simulink model "npc_controller"  (R2022a)
settings: Solver=FixedStepDiscrete  StartTime=0.0  StopTime=20  RelTol=1e-3  EnableMultiTasking=on
undefined symbols (not defined in the file): CAN_O_INT, CANA_BASE, Down, GPTRIP1SEL, GPTRIP2SEL, GPTRIP3SEL, Tsw, TZ1, TZ2, TZ3, Up, V2G_en
libraries: simulink x171, hdlsllib x90, c2802xlib x46, c2837xDlib x19, c280xlib x12, canmsglib x9, c2838xlib x8, idelinklib_common x5, c2806xlib x2, slpidlib x2, c28004xlib x2, c281xlib x2
(part 50 of 55)

== system npc_controller/IDLE_AND_TIMER/codegen/CAN_Task/Tx_Handler/Run Tx Routine/TxStatusData/Tx Pri2 ID131 ==
  Action Port : ActionPort  ActionPortLabel=case [ 2 ]:
  CAN Pack1 : canmsglib/CAN Pack  MsgList=(none)  MsgName=CAN Msg  MsgIDType=Standard (11-bit identifier)  MsgIdentifier=0x131  MsgLength=8  Remote=off  ApplyMinMax=off  BusOutput=off  SignalInfo={}
      settings: SourceProductBaseCode=XP,ME,VN  DataFormat=raw data
  Constant1 : Constant  Value=3  OutDataTypeStr=uint8
  Constant2 : Constant  Value=0.1  OutDataTypeStr=single
  Constant3 : Constant  Value=0.01  OutDataTypeStr=single
  Constant4 : Constant  Value=0.01  OutDataTypeStr=single
  Constant5 : Constant  Value=0.1  OutDataTypeStr=single
  Data Store Read1 : DataStoreRead  DataStoreName=f32VinB  IndexOptions=Index vector (dialog)  Indices=1  OutputSizes=1
  Data Store Read2 : DataStoreRead  DataStoreName=f32VinC  IndexOptions=Index vector (dialog)  Indices=1  OutputSizes=1
  Data Store Read4 : DataStoreRead  DataStoreName=f32IinB  IndexOptions=Index vector (dialog)  Indices=1  OutputSizes=1
  Data Store Read5 : DataStoreRead  DataStoreName=f32IinC  IndexOptions=Index vector (dialog)  Indices=1  OutputSizes=1
  Data Store Write1 : DataStoreWrite  DataStoreName=u8CanTxIndex  IndexOptions=Index vector (dialog)  Indices=1  OutputSizes=1
  Float Data to Bytes : Subsystem
  Float Data to Bytes1 : Subsystem
  Float Data to Bytes2 : Subsystem
  Float Data to Bytes3 : Subsystem
  Vector Concatenate : Concatenate  NumInputs=8
  eCAN Transmit : c280xlib/eCAN Transmit  chipFamily=C280x  useModule=eCAN_A  mailboxNo=2  messageID=hex2dec('0131')  messageType=Standard (11-bit identifier)  enableBlockingMode=off  postInterrupt=off  interruptLine=0
      settings: SourceProductBaseCode=TIC2000
  wires:
  Constant1/1 -> Data Store Write1/1
  Data Store Read4/1 -> Float Data to Bytes1/1(Float Data)
  Data Store Read2/1 -> Float Data to Bytes/1(Float Data)
  Constant2/1 -> Float Data to Bytes/2(Resol.)
  CAN Pack1/1 -> eCAN Transmit/1
  Float Data to Bytes/1(u8Lsb) -> Vector Concatenate/3
  Float Data to Bytes3/1(u8Lsb) -> Vector Concatenate/1
  Float Data to Bytes3/2(u8Msb) -> Vector Concatenate/2
  Float Data to Bytes2/2(u8Msb) -> Vector Concatenate/8
  Constant4/1 -> Float Data to Bytes2/2(Resol.)
  Float Data to Bytes2/1(u8Lsb) -> Vector Concatenate/7
  Data Store Read5/1 -> Float Data to Bytes2/1(Float Data)
  Float Data to Bytes/2(u8Msb) -> Vector Concatenate/4
  Data Store Read1/1 -> Float Data to Bytes3/1(Float Data)
  Float Data to Bytes1/1(u8Lsb) -> Vector Concatenate/5
  Vector Concatenate/1 -> CAN Pack1/1
  Constant3/1 -> Float Data to Bytes1/2(Resol.)
  Float Data to Bytes1/2(u8Msb) -> Vector Concatenate/6
  Constant5/1 -> Float Data to Bytes3/2(Resol.)

== system npc_controller/IDLE_AND_TIMER/codegen/CAN_Task/Tx_Handler/Run Tx Routine/TxStatusData/Tx Pri3 ID132 ==
  Action Port : ActionPort  ActionPortLabel=case [ 3 ]:
  CAN Pack1 : canmsglib/CAN Pack  MsgList=(none)  MsgName=CAN Msg  MsgIDType=Standard (11-bit identifier)  MsgIdentifier=0x132  MsgLength=8  Remote=off  ApplyMinMax=off  BusOutput=off  SignalInfo={}
      settings: SourceProductBaseCode=XP,ME,VN  DataFormat=raw data
  Constant1 : Constant  Value=4  OutDataTypeStr=uint8
  Constant2 : Constant  Value=0.01  OutDataTypeStr=single
  Constant3 : Constant  Value=0.01  OutDataTypeStr=single
  Constant4 : Constant  Value=0.1  OutDataTypeStr=single
  Constant5 : Constant  Value=0.01  OutDataTypeStr=single
  Data Store Read1 : DataStoreRead  DataStoreName=f32IphaseA  IndexOptions=Index vector (dialog)  Indices=1  OutputSizes=1
  Data Store Read2 : DataStoreRead  DataStoreName=f32IphaseB  IndexOptions=Index vector (dialog)  Indices=1  OutputSizes=1
  Data Store Read4 : DataStoreRead  DataStoreName=f32IphaseC  IndexOptions=Index vector (dialog)  Indices=1  OutputSizes=1
  Data Store Read5 : DataStoreRead  DataStoreName=f32Vpfc  IndexOptions=Index vector (dialog)  Indices=1  OutputSizes=1
  Data Store Write1 : DataStoreWrite  DataStoreName=u8CanTxIndex  IndexOptions=Index vector (dialog)  Indices=1  OutputSizes=1
  Float Data to Bytes : Subsystem
  Float Data to Bytes1 : Subsystem
  Float Data to Bytes2 : Subsystem
  Float Data to Bytes3 : Subsystem
  Vector Concatenate : Concatenate  NumInputs=8
  eCAN Transmit : c280xlib/eCAN Transmit  chipFamily=C280x  useModule=eCAN_A  mailboxNo=2  messageID=hex2dec('0132')  messageType=Standard (11-bit identifier)  enableBlockingMode=off  postInterrupt=off  interruptLine=0
      settings: SourceProductBaseCode=TIC2000
  wires:
  Constant5/1 -> Float Data to Bytes3/2(Resol.)
  Float Data to Bytes1/2(u8Msb) -> Vector Concatenate/6
  Constant3/1 -> Float Data to Bytes1/2(Resol.)
  Vector Concatenate/1 -> CAN Pack1/1
  Float Data to Bytes1/1(u8Lsb) -> Vector Concatenate/5
  Data Store Read1/1 -> Float Data to Bytes3/1(Float Data)
  Float Data to Bytes/2(u8Msb) -> Vector Concatenate/4
  Data Store Read5/1 -> Float Data to Bytes2/1(Float Data)
  Float Data to Bytes2/1(u8Lsb) -> Vector Concatenate/7
  Constant4/1 -> Float Data to Bytes2/2(Resol.)
  Float Data to Bytes2/2(u8Msb) -> Vector Concatenate/8
  Float Data to Bytes3/2(u8Msb) -> Vector Concatenate/2
  Float Data to Bytes3/1(u8Lsb) -> Vector Concatenate/1
  Float Data to Bytes/1(u8Lsb) -> Vector Concatenate/3
  CAN Pack1/1 -> eCAN Transmit/1
  Constant2/1 -> Float Data to Bytes/2(Resol.)
  Data Store Read2/1 -> Float Data to Bytes/1(Float Data)
  Data Store Read4/1 -> Float Data to Bytes1/1(Float Data)
  Constant1/1 -> Data Store Write1/1

== system npc_controller/IDLE_AND_TIMER/codegen/CAN_Task/Tx_Handler/Run Tx Routine/TxStatusData/Tx Pri4 ID133 ==
  Action Port : ActionPort  ActionPortLabel=case [ 4 ]:
  CAN Pack1 : canmsglib/CAN Pack  MsgList=(none)  MsgName=CAN Msg  MsgIDType=Standard (11-bit identifier)  MsgIdentifier=0x133  MsgLength=8  Remote=off  ApplyMinMax=off  BusOutput=off  SignalInfo={}
      settings: SourceProductBaseCode=XP,ME,VN  DataFormat=raw data
  Constant1 : Constant  Value=0  OutDataTypeStr=uint8
  Constant2 : Constant  Value=0  OutDataTypeStr=uint8
  Data Store Read1 : DataStoreRead  DataStoreName=u8TnpcA  IndexOptions=Index vector (dialog)  Indices=1  OutputSizes=1
  Data Store Read2 : DataStoreRead  DataStoreName=u8TnpcC  IndexOptions=Index vector (dialog)  Indices=1  OutputSizes=1
  Data Store Read3 : DataStoreRead  DataStoreName=u8TnpcB  IndexOptions=Index vector (dialog)  Indices=1  OutputSizes=1
  Data Store Read4 : DataStoreRead  DataStoreName=u8TclllcP2  IndexOptions=Index vector (dialog)  Indices=1  OutputSizes=1
  Data Store Read6 : DataStoreRead  DataStoreName=u8TclllcP1  IndexOptions=Index vector (dialog)  Indices=1  OutputSizes=1
  Data Store Write1 : DataStoreWrite  DataStoreName=u8CanTxIndex  IndexOptions=Index vector (dialog)  Indices=1  OutputSizes=1
  Vector Concatenate : Concatenate  NumInputs=8
  eCAN Transmit : c280xlib/eCAN Transmit  chipFamily=C280x  useModule=eCAN_A  mailboxNo=3  messageID=hex2dec('0133')  messageType=Standard (11-bit identifier)  enableBlockingMode=off  postInterrupt=off  interruptLine=0
      settings: SourceProductBaseCode=TIC2000
  wires:
  Constant1/1 -> Data Store Write1/1
  CAN Pack1/1 -> eCAN Transmit/1
  Data Store Read1/1 -> Vector Concatenate/1
  Data Store Read3/1 -> Vector Concatenate/2
  Vector Concatenate/1 -> CAN Pack1/1
  Data Store Read6/1 -> Vector Concatenate/4
  Data Store Read2/1 -> Vector Concatenate/3
  Data Store Read4/1 -> Vector Concatenate/5
  Constant2/1 -> Vector Concatenate/6, Vector Concatenate/7, Vector Concatenate/8

== system npc_controller/IDLE_AND_TIMER/codegen/IDLE/idle_task/hkeep/tfv/hkeep1/HKEEP.tfvIphaseA ==
  input : Inport  OutDataTypeStr=uint16  PortDimensions=1
  assert_lim : Inport  Port=2  OutDataTypeStr=uint16  PortDimensions=1
  assert_vld : Inport  Port=3  OutDataTypeStr=uint16  PortDimensions=1
  deassert_lim : Inport  Port=4  OutDataTypeStr=uint16  PortDimensions=1
  deassert_vld : Inport  Port=5  OutDataTypeStr=uint16  PortDimensions=1
  f : TriggerPort  TriggerType=function-call  VariantControl=(inherit)
      settings: CopyFcn=Stateflow.SLINSF.SimulinkMan.removeBlockPreDeleteFcn  PreDeleteFcn=Stateflow.SLINSF.SimulinkMan.unsafePredeleteFcn
  Data Store Read : DataStoreRead  DataStoreName=cnt_1ms  IndexOptions=Index vector (dialog)  Indices=1  OutputSizes=1
  Data Type Conversion : DataTypeConversion  OutDataTypeStr=boolean  SaturateOnIntegerOverflow=off  RndMeth=Floor
  MATLAB System : MATLABSystem  System=tfv_latch  SimulateUsing=Code generation
      mask Type: tfv_latch
      mask Display:
      | disp('tfv_latch');
      | port_label('input',1,'input');
      | port_label('input',2,'assert_lim');
      | port_label('input',3,'assert_vld');
      | port_label('input',4,'deassert_lim');
      | port_label('input',5,'deassert_vld');
      | port_label('input',6,'tmr');
      | port_label('output',1,'status');
  tfv_iphasaea : Outport  OutDataTypeStr=boolean
  wires:
  Data Type Conversion/1 -> tfv_iphasaea/1
  Data Store Read/1 -> MATLAB System/6
  deassert_vld/1 -> MATLAB System/5
  deassert_lim/1 -> MATLAB System/4
  assert_vld/1 -> MATLAB System/3
  assert_lim/1 -> MATLAB System/2
  input/1 -> MATLAB System/1
  MATLAB System/1 -> Data Type Conversion/1

== system npc_controller/IDLE_AND_TIMER/codegen/IDLE/idle_task/hkeep/tfv/hkeep1/HKEEP.tfvIphaseB ==
  input : Inport  OutDataTypeStr=uint16  PortDimensions=1
  assert_lim : Inport  Port=2  OutDataTypeStr=uint16  PortDimensions=1
  assert_vld : Inport  Port=3  OutDataTypeStr=uint16  PortDimensions=1
  deassert_lim : Inport  Port=4  OutDataTypeStr=uint16  PortDimensions=1
  deassert_vld : Inport  Port=5  OutDataTypeStr=uint16  PortDimensions=1
  f : TriggerPort  TriggerType=function-call  VariantControl=(inherit)
      settings: CopyFcn=Stateflow.SLINSF.SimulinkMan.removeBlockPreDeleteFcn  PreDeleteFcn=Stateflow.SLINSF.SimulinkMan.unsafePredeleteFcn
  Data Store Read : DataStoreRead  DataStoreName=cnt_1ms  IndexOptions=Index vector (dialog)  Indices=1  OutputSizes=1
  Data Type Conversion : DataTypeConversion  OutDataTypeStr=boolean  SaturateOnIntegerOverflow=off  RndMeth=Floor
  MATLAB System : MATLABSystem  System=tfv_latch  SimulateUsing=Code generation
      mask Type: tfv_latch
      mask Display:
      | disp('tfv_latch');
      | port_label('input',1,'input');
      | port_label('input',2,'assert_lim');
      | port_label('input',3,'assert_vld');
      | port_label('input',4,'deassert_lim');
      | port_label('input',5,'deassert_vld');
      | port_label('input',6,'tmr');
      | port_label('output',1,'status');
  tfv_iphaseb : Outport  OutDataTypeStr=boolean
  wires:
  Data Type Conversion/1 -> tfv_iphaseb/1
  Data Store Read/1 -> MATLAB System/6
  deassert_vld/1 -> MATLAB System/5
  deassert_lim/1 -> MATLAB System/4
  assert_vld/1 -> MATLAB System/3
  assert_lim/1 -> MATLAB System/2
  input/1 -> MATLAB System/1
  MATLAB System/1 -> Data Type Conversion/1

== system npc_controller/IDLE_AND_TIMER/codegen/IDLE/idle_task/hkeep/tfv/hkeep1/HKEEP.tfvIphaseC ==
  input : Inport  OutDataTypeStr=uint16  PortDimensions=1
  assert_lim : Inport  Port=2  OutDataTypeStr=uint16  PortDimensions=1
  assert_vld : Inport  Port=3  OutDataTypeStr=uint16  PortDimensions=1
  deassert_lim : Inport  Port=4  OutDataTypeStr=uint16  PortDimensions=1
  deassert_vld : Inport  Port=5  OutDataTypeStr=uint16  PortDimensions=1
  f : TriggerPort  TriggerType=function-call  VariantControl=(inherit)
      settings: CopyFcn=Stateflow.SLINSF.SimulinkMan.removeBlockPreDeleteFcn  PreDeleteFcn=Stateflow.SLINSF.SimulinkMan.unsafePredeleteFcn
  Data Store Read : DataStoreRead  DataStoreName=cnt_1ms  IndexOptions=Index vector (dialog)  Indices=1  OutputSizes=1
  Data Type Conversion : DataTypeConversion  OutDataTypeStr=boolean  SaturateOnIntegerOverflow=off  RndMeth=Floor
  MATLAB System : MATLABSystem  System=tfv_latch  SimulateUsing=Code generation
      mask Type: tfv_latch
      mask Display:
      | disp('tfv_latch');
      | port_label('input',1,'input');
      | port_label('input',2,'assert_lim');
      | port_label('input',3,'assert_vld');
      | port_label('input',4,'deassert_lim');
      | port_label('input',5,'deassert_vld');
      | port_label('input',6,'tmr');
      | port_label('output',1,'status');
  tfv_iphasec : Outport  OutDataTypeStr=boolean
  wires:
  Data Type Conversion/1 -> tfv_iphasec/1
  Data Store Read/1 -> MATLAB System/6
  deassert_vld/1 -> MATLAB System/5
  deassert_lim/1 -> MATLAB System/4
  assert_vld/1 -> MATLAB System/3
  assert_lim/1 -> MATLAB System/2
  input/1 -> MATLAB System/1
  MATLAB System/1 -> Data Type Conversion/1

== system npc_controller/IDLE_AND_TIMER/codegen/IDLE/idle_task/hkeep/tfv/hkeep1/HKEEP.tfvVa ==
  input : Inport  OutDataTypeStr=uint16  PortDimensions=1
  assert_lim : Inport  Port=2  OutDataTypeStr=uint16  PortDimensions=1
  assert_vld : Inport  Port=3  OutDataTypeStr=uint16  PortDimensions=1
  deassert_lim : Inport  Port=4  OutDataTypeStr=uint16  PortDimensions=1
  deassert_vld : Inport  Port=5  OutDataTypeStr=uint16  PortDimensions=1
  f : TriggerPort  TriggerType=function-call  VariantControl=(inherit)
      settings: CopyFcn=Stateflow.SLINSF.SimulinkMan.removeBlockPreDeleteFcn  PreDeleteFcn=Stateflow.SLINSF.SimulinkMan.unsafePredeleteFcn
  Data Store Read : DataStoreRead  DataStoreName=cnt_1ms  IndexOptions=Index vector (dialog)  Indices=1  OutputSizes=1
  Data Type Conversion : DataTypeConversion  OutDataTypeStr=boolean  SaturateOnIntegerOverflow=off  RndMeth=Floor
  MATLAB System : MATLABSystem  System=tfv_latch  SimulateUsing=Code generation
      mask Type: tfv_latch
      mask Display:
      | disp('tfv_latch');
      | port_label('input',1,'input');
      | port_label('input',2,'assert_lim');
      | port_label('input',3,'assert_vld');
      | port_label('input',4,'deassert_lim');
      | port_label('input',5,'deassert_vld');
      | port_label('input',6,'tmr');
      | port_label('output',1,'status');
  tfv_va : Outport  OutDataTypeStr=boolean
  wires:
  Data Type Conversion/1 -> tfv_va/1
  Data Store Read/1 -> MATLAB System/6
  deassert_vld/1 -> MATLAB System/5
  deassert_lim/1 -> MATLAB System/4
  assert_vld/1 -> MATLAB System/3
  assert_lim/1 -> MATLAB System/2
  input/1 -> MATLAB System/1
  MATLAB System/1 -> Data Type Conversion/1

== system npc_controller/IDLE_AND_TIMER/codegen/IDLE/idle_task/hkeep/tfv/hkeep1/HKEEP.tfvVaux ==
  input : Inport  OutDataTypeStr=uint16  PortDimensions=1
  assert_lim : Inport  Port=2  OutDataTypeStr=uint16  PortDimensions=1
  assert_vld : Inport  Port=3  OutDataTypeStr=uint16  PortDimensions=1
  deassert_lim : Inport  Port=4  OutDataTypeStr=uint16  PortDimensions=1
  deassert_vld : Inport  Port=5  OutDataTypeStr=uint16  PortDimensions=1
  f : TriggerPort  TriggerType=function-call  VariantControl=(inherit)
      settings: CopyFcn=Stateflow.SLINSF.SimulinkMan.removeBlockPreDeleteFcn  PreDeleteFcn=Stateflow.SLINSF.SimulinkMan.unsafePredeleteFcn
  Data Store Read : DataStoreRead  DataStoreName=cnt_1ms  IndexOptions=Index vector (dialog)  Indices=1  OutputSizes=1
  Data Type Conversion : DataTypeConversion  OutDataTypeStr=boolean  SaturateOnIntegerOverflow=off  RndMeth=Floor
  MATLAB System : MATLABSystem  System=tfv_latch  SimulateUsing=Code generation
      mask Type: tfv_latch
      mask Display:
      | disp('tfv_latch');
      | port_label('input',1,'input');
      | port_label('input',2,'assert_lim');
      | port_label('input',3,'assert_vld');
      | port_label('input',4,'deassert_lim');
      | port_label('input',5,'deassert_vld');
      | port_label('input',6,'tmr');
      | port_label('output',1,'status');
  Rate Transition2 : RateTransition  Commented=on
  tfv_vaux : Outport  OutDataTypeStr=boolean
  wires:
  Data Type Conversion/1 -> tfv_vaux/1
  deassert_vld/1 -> MATLAB System/5
  deassert_lim/1 -> MATLAB System/4
  assert_vld/1 -> MATLAB System/3
  assert_lim/1 -> MATLAB System/2
  input/1 -> MATLAB System/1
  MATLAB System/1 -> Data Type Conversion/1
  Data Store Read/1 -> MATLAB System/6

== system npc_controller/IDLE_AND_TIMER/codegen/IDLE/idle_task/hkeep/tfv/hkeep1/HKEEP.tfvVb ==
  input : Inport  OutDataTypeStr=uint16  PortDimensions=1
  assert_lim : Inport  Port=2  OutDataTypeStr=uint16  PortDimensions=1
  assert_vld : Inport  Port=3  OutDataTypeStr=uint16  PortDimensions=1
  deassert_lim : Inport  Port=4  OutDataTypeStr=uint16  PortDimensions=1
  deassert_vld : Inport  Port=5  OutDataTypeStr=uint16  PortDimensions=1
  f : TriggerPort  TriggerType=function-call  VariantControl=(inherit)
      settings: CopyFcn=Stateflow.SLINSF.SimulinkMan.removeBlockPreDeleteFcn  PreDeleteFcn=Stateflow.SLINSF.SimulinkMan.unsafePredeleteFcn
  Data Store Read : DataStoreRead  DataStoreName=cnt_1ms  IndexOptions=Index vector (dialog)  Indices=1  OutputSizes=1
  Data Type Conversion : DataTypeConversion  OutDataTypeStr=boolean  SaturateOnIntegerOverflow=off  RndMeth=Floor
  MATLAB System : MATLABSystem  System=tfv_latch  SimulateUsing=Code generation
      mask Type: tfv_latch
      mask Display:
      | disp('tfv_latch');
      | port_label('input',1,'input');
      | port_label('input',2,'assert_lim');
      | port_label('input',3,'assert_vld');
      | port_label('input',4,'deassert_lim');
      | port_label('input',5,'deassert_vld');
      | port_label('input',6,'tmr');
      | port_label('output',1,'status');
  tfv_vb : Outport  OutDataTypeStr=boolean
  wires:
  Data Type Conversion/1 -> tfv_vb/1
  Data Store Read/1 -> MATLAB System/6
  deassert_vld/1 -> MATLAB System/5
  deassert_lim/1 -> MATLAB System/4
  assert_vld/1 -> MATLAB System/3
  assert_lim/1 -> MATLAB System/2
  input/1 -> MATLAB System/1
  MATLAB System/1 -> Data Type Conversion/1

== system npc_controller/IDLE_AND_TIMER/codegen/IDLE/idle_task/hkeep/tfv/hkeep1/HKEEP.tfvVbulk ==
  input : Inport  OutDataTypeStr=uint16  PortDimensions=1
  assert_lim : Inport  Port=2  OutDataTypeStr=uint16  PortDimensions=1
  assert_vld : Inport  Port=3  OutDataTypeStr=uint16  PortDimensions=1
  deassert_lim : Inport  Port=4  OutDataTypeStr=uint16  PortDimensions=1
  deassert_vld : Inport  Port=5  OutDataTypeStr=uint16  PortDimensions=1
  f : TriggerPort  TriggerType=function-call  VariantControl=(inherit)
      settings: CopyFcn=Stateflow.SLINSF.SimulinkMan.removeBlockPreDeleteFcn  PreDeleteFcn=Stateflow.SLINSF.SimulinkMan.unsafePredeleteFcn
  Data Store Read : DataStoreRead  DataStoreName=cnt_1ms  IndexOptions=Index vector (dialog)  Indices=1  OutputSizes=1
  Data Type Conversion : DataTypeConversion  OutDataTypeStr=boolean  SaturateOnIntegerOverflow=off  RndMeth=Floor
  MATLAB System : MATLABSystem  System=tfv_latch  SimulateUsing=Code generation
      mask Type: tfv_latch
      mask Display:
      | disp('tfv_latch');
      | port_label('input',1,'input');
      | port_label('input',2,'assert_lim');
      | port_label('input',3,'assert_vld');
      | port_label('input',4,'deassert_lim');
      | port_label('input',5,'deassert_vld');
      | port_label('input',6,'tmr');
      | port_label('output',1,'status');
  tfv_vbulk : Outport  OutDataTypeStr=boolean
  wires:
  Data Type Conversion/1 -> tfv_vbulk/1
  Data Store Read/1 -> MATLAB System/6
  deassert_vld/1 -> MATLAB System/5
  deassert_lim/1 -> MATLAB System/4
  assert_vld/1 -> MATLAB System/3
  assert_lim/1 -> MATLAB System/2
  input/1 -> MATLAB System/1
  MATLAB System/1 -> Data Type Conversion/1

== system npc_controller/IDLE_AND_TIMER/codegen/IDLE/idle_task/hkeep/tfv/hkeep1/HKEEP.tfvVc ==
  input : Inport  OutDataTypeStr=uint16  PortDimensions=1
  assert_lim : Inport  Port=2  OutDataTypeStr=uint16  PortDimensions=1
  assert_vld : Inport  Port=3  OutDataTypeStr=uint16  PortDimensions=1
  deassert_lim : Inport  Port=4  OutDataTypeStr=uint16  PortDimensions=1
  deassert_vld : Inport  Port=5  OutDataTypeStr=uint16  PortDimensions=1
  f : TriggerPort  TriggerType=function-call  VariantControl=(inherit)
      settings: CopyFcn=Stateflow.SLINSF.SimulinkMan.removeBlockPreDeleteFcn  PreDeleteFcn=Stateflow.SLINSF.SimulinkMan.unsafePredeleteFcn
  Data Store Read : DataStoreRead  DataStoreName=cnt_1ms  IndexOptions=Index vector (dialog)  Indices=1  OutputSizes=1
  Data Type Conversion : DataTypeConversion  OutDataTypeStr=boolean  SaturateOnIntegerOverflow=off  RndMeth=Floor
  MATLAB System : MATLABSystem  System=tfv_latch  SimulateUsing=Code generation
      mask Type: tfv_latch
      mask Display:
      | disp('tfv_latch');
      | port_label('input',1,'input');
      | port_label('input',2,'assert_lim');
      | port_label('input',3,'assert_vld');
      | port_label('input',4,'deassert_lim');
      | port_label('input',5,'deassert_vld');
      | port_label('input',6,'tmr');
      | port_label('output',1,'status');
  tfv_vc : Outport  OutDataTypeStr=boolean
  wires:
  Data Type Conversion/1 -> tfv_vc/1
  Data Store Read/1 -> MATLAB System/6
  deassert_vld/1 -> MATLAB System/5
  deassert_lim/1 -> MATLAB System/4
  assert_vld/1 -> MATLAB System/3
  assert_lim/1 -> MATLAB System/2
  input/1 -> MATLAB System/1
  MATLAB System/1 -> Data Type Conversion/1

== system npc_controller/IDLE_AND_TIMER/codegen/IDLE/idle_task/hkeep/tfv/hkeep1/HKEEP.tfvVmid ==
  input : Inport  OutDataTypeStr=uint16  PortDimensions=1
  assert_lim : Inport  Port=2  OutDataTypeStr=uint16  PortDimensions=1
  assert_vld : Inport  Port=3  OutDataTypeStr=uint16  PortDimensions=1
  deassert_lim : Inport  Port=4  OutDataTypeStr=uint16  PortDimensions=1
  deassert_vld : Inport  Port=5  OutDataTypeStr=uint16  PortDimensions=1
  f : TriggerPort  TriggerType=function-call  VariantControl=(inherit)
      settings: CopyFcn=Stateflow.SLINSF.SimulinkMan.removeBlockPreDeleteFcn  PreDeleteFcn=Stateflow.SLINSF.SimulinkMan.unsafePredeleteFcn
  Data Store Read : DataStoreRead  DataStoreName=cnt_1ms  IndexOptions=Index vector (dialog)  Indices=1  OutputSizes=1
  Data Type Conversion : DataTypeConversion  OutDataTypeStr=boolean  SaturateOnIntegerOverflow=off  RndMeth=Floor
  MATLAB System : MATLABSystem  System=tfv_latch  SimulateUsing=Code generation
      mask Type: tfv_latch
      mask Display:
      | disp('tfv_latch');
      | port_label('input',1,'input');
      | port_label('input',2,'assert_lim');
      | port_label('input',3,'assert_vld');
      | port_label('input',4,'deassert_lim');
      | port_label('input',5,'deassert_vld');
      | port_label('input',6,'tmr');
      | port_label('output',1,'status');
  Rate Transition2 : RateTransition  Commented=on
  tfv_vmid : Outport  OutDataTypeStr=boolean
  wires:
  Data Type Conversion/1 -> tfv_vmid/1
  deassert_vld/1 -> MATLAB System/5
  deassert_lim/1 -> MATLAB System/4
  assert_vld/1 -> MATLAB System/3
  assert_lim/1 -> MATLAB System/2
  input/1 -> MATLAB System/1
  MATLAB System/1 -> Data Type Conversion/1
  Data Store Read/1 -> MATLAB System/6

== system npc_controller/IDLE_AND_TIMER/codegen/IDLE/idle_task/hkeep/tz/System Outputs2 ==

== system npc_controller/IDLE_AND_TIMER/codegen/IDLE/idle_task/hkeep/tz1/System Outputs2 ==

== system npc_controller/IDLE_AND_TIMER/codegen/IDLE/idle_task/set_tmp_mux/incr_cnt_tmp_mux/cnt_idle ==
  Action Port : ActionPort  ActionPortLabel=if(u1 < 4)
  Add : Sum
  Constant : Constant  OutDataTypeStr=uint16
  Data Store Read1 : DataStoreRead  DataStoreName=cnt_tmp_mux  IndexOptions=Index vector (dialog)  Indices=1  OutputSizes=1
  Data Store Write : DataStoreWrite  DataStoreName=cnt_tmp_mux  IndexOptions=Index vector (dialog)  Indices=1  OutputSizes=1
  wires:
  Data Store Read1/1 -> Add/1
  Add/1 -> Data Store Write/1
  Constant/1 -> Add/2

== system npc_controller/IDLE_AND_TIMER/codegen/IDLE/idle_task/set_tmp_mux/incr_cnt_tmp_mux/cnt_idle_sat ==
  Action Port : ActionPort  ActionPortLabel=else
  Constant : Constant  Value=0  OutDataTypeStr=uint16
  Data Store Write : DataStoreWrite  DataStoreName=cnt_tmp_mux  IndexOptions=Index vector (dialog)  Indices=1  OutputSizes=1
  wires:
  Constant/1 -> Data Store Write/1

== system npc_controller/IDLE_AND_TIMER/codegen/IDLE/idle_task/set_tmp_mux/parse_cnt_tmp_mux/cnt_tmp_mux_0 ==
  Action Port : ActionPort  ActionPortLabel=case [ 0 ]:
  Constant : Constant  Value=0  OutDataTypeStr=boolean  SampleTime=-1
  Constant1 : Constant  Value=0  OutDataTypeStr=boolean  SampleTime=-1
  Constant2 : Constant  Value=0  OutDataTypeStr=boolean  SampleTime=-1
  Data Store Write : DataStoreWrite  DataStoreName=tmp_mux_s0  IndexOptions=Index vector (dialog)  Indices=1  OutputSizes=1
  Data Store Write1 : DataStoreWrite  DataStoreName=tmp_mux_s1  IndexOptions=Index vector (dialog)  Indices=1  OutputSizes=1
  Data Store Write2 : DataStoreWrite  DataStoreName=tmp_mux_s2  IndexOptions=Index vector (dialog)  Indices=1  OutputSizes=1
  wires:
  Constant/1 -> Data Store Write/1
  Constant1/1 -> Data Store Write1/1
  Constant2/1 -> Data Store Write2/1

== system npc_controller/IDLE_AND_TIMER/codegen/IDLE/idle_task/set_tmp_mux/parse_cnt_tmp_mux/cnt_tmp_mux_1 ==
  Action Port : ActionPort  ActionPortLabel=case [ 1 ]:
  Constant : Constant  OutDataTypeStr=boolean  SampleTime=-1
  Constant1 : Constant  Value=0  OutDataTypeStr=boolean  SampleTime=-1
  Constant2 : Constant  Value=0  OutDataTypeStr=boolean  SampleTime=-1
  Data Store Write : DataStoreWrite  DataStoreName=tmp_mux_s0  IndexOptions=Index vector (dialog)  Indices=1  OutputSizes=1
  Data Store Write1 : DataStoreWrite  DataStoreName=tmp_mux_s1  IndexOptions=Index vector (dialog)  Indices=1  OutputSizes=1
  Data Store Write2 : DataStoreWrite  DataStoreName=tmp_mux_s2  IndexOptions=Index vector (dialog)  Indices=1  OutputSizes=1
  wires:
  Constant2/1 -> Data Store Write2/1
  Constant1/1 -> Data Store Write1/1
  Constant/1 -> Data Store Write/1

== system npc_controller/IDLE_AND_TIMER/codegen/IDLE/idle_task/set_tmp_mux/parse_cnt_tmp_mux/cnt_tmp_mux_2 ==
  Action Port : ActionPort  ActionPortLabel=case [ 2 ]:
  Constant : Constant  Value=0  OutDataTypeStr=boolean  SampleTime=-1
  Constant1 : Constant  OutDataTypeStr=boolean  SampleTime=-1
  Constant2 : Constant  Value=0  OutDataTypeStr=boolean  SampleTime=-1
  Data Store Write : DataStoreWrite  DataStoreName=tmp_mux_s0  IndexOptions=Index vector (dialog)  Indices=1  OutputSizes=1
  Data Store Write1 : DataStoreWrite  DataStoreName=tmp_mux_s1  IndexOptions=Index vector (dialog)  Indices=1  OutputSizes=1
  Data Store Write2 : DataStoreWrite  DataStoreName=tmp_mux_s2  IndexOptions=Index vector (dialog)  Indices=1  OutputSizes=1
  wires:
  Constant/1 -> Data Store Write/1
  Constant1/1 -> Data Store Write1/1
  Constant2/1 -> Data Store Write2/1

== system npc_controller/IDLE_AND_TIMER/codegen/IDLE/idle_task/set_tmp_mux/parse_cnt_tmp_mux/cnt_tmp_mux_3 ==
  Action Port : ActionPort  ActionPortLabel=case [ 3 ]:
  Constant : Constant  OutDataTypeStr=boolean  SampleTime=-1
  Constant1 : Constant  OutDataTypeStr=boolean  SampleTime=-1
  Constant2 : Constant  Value=0  OutDataTypeStr=boolean  SampleTime=-1
  Data Store Write : DataStoreWrite  DataStoreName=tmp_mux_s0  IndexOptions=Index vector (dialog)  Indices=1  OutputSizes=1
  Data Store Write1 : DataStoreWrite  DataStoreName=tmp_mux_s1  IndexOptions=Index vector (dialog)  Indices=1  OutputSizes=1
  Data Store Write2 : DataStoreWrite  DataStoreName=tmp_mux_s2  IndexOptions=Index vector (dialog)  Indices=1  OutputSizes=1
  wires:
  Constant2/1 -> Data Store Write2/1
  Constant1/1 -> Data Store Write1/1
  Constant/1 -> Data Store Write/1

== system npc_controller/IDLE_AND_TIMER/codegen/IDLE/idle_task1/hkeep/tfv/hkeep1/HKEEP.tfvIphaseA ==
  input : Inport  OutDataTypeStr=uint16  PortDimensions=1
  assert_lim : Inport  Port=2  OutDataTypeStr=uint16  PortDimensions=1
  assert_vld : Inport  Port=3  OutDataTypeStr=uint16  PortDimensions=1
  deassert_lim : Inport  Port=4  OutDataTypeStr=uint16  PortDimensions=1
  deassert_vld : Inport  Port=5  OutDataTypeStr=uint16  PortDimensions=1
  f : TriggerPort  TriggerType=function-call  VariantControl=(inherit)
      settings: CopyFcn=Stateflow.SLINSF.SimulinkMan.removeBlockPreDeleteFcn  PreDeleteFcn=Stateflow.SLINSF.SimulinkMan.unsafePredeleteFcn
  Data Store Read : DataStoreRead  DataStoreName=cnt_1ms  IndexOptions=Index vector (dialog)  Indices=1  OutputSizes=1
  Data Type Conversion : DataTypeConversion  OutDataTypeStr=boolean  SaturateOnIntegerOverflow=off  RndMeth=Floor
  MATLAB System : MATLABSystem  System=tfv_latch  SimulateUsing=Code generation
      mask Type: tfv_latch
      mask Display:
      | disp('tfv_latch');
      | port_label('input',1,'input');
      | port_label('input',2,'assert_lim');
      | port_label('input',3,'assert_vld');
      | port_label('input',4,'deassert_lim');
      | port_label('input',5,'deassert_vld');
      | port_label('input',6,'tmr');
      | port_label('output',1,'status');
  tfv_iphasaea : Outport  OutDataTypeStr=boolean
  wires:
  Data Type Conversion/1 -> tfv_iphasaea/1
  Data Store Read/1 -> MATLAB System/6
  deassert_vld/1 -> MATLAB System/5
  deassert_lim/1 -> MATLAB System/4
  assert_vld/1 -> MATLAB System/3
  assert_lim/1 -> MATLAB System/2
  input/1 -> MATLAB System/1
  MATLAB System/1 -> Data Type Conversion/1

== system npc_controller/IDLE_AND_TIMER/codegen/IDLE/idle_task1/hkeep/tfv/hkeep1/HKEEP.tfvIphaseB ==
  input : Inport  OutDataTypeStr=uint16  PortDimensions=1
  assert_lim : Inport  Port=2  OutDataTypeStr=uint16  PortDimensions=1
  assert_vld : Inport  Port=3  OutDataTypeStr=uint16  PortDimensions=1
  deassert_lim : Inport  Port=4  OutDataTypeStr=uint16  PortDimensions=1
  deassert_vld : Inport  Port=5  OutDataTypeStr=uint16  PortDimensions=1
  f : TriggerPort  TriggerType=function-call  VariantControl=(inherit)
      settings: CopyFcn=Stateflow.SLINSF.SimulinkMan.removeBlockPreDeleteFcn  PreDeleteFcn=Stateflow.SLINSF.SimulinkMan.unsafePredeleteFcn
  Data Store Read : DataStoreRead  DataStoreName=cnt_1ms  IndexOptions=Index vector (dialog)  Indices=1  OutputSizes=1
  Data Type Conversion : DataTypeConversion  OutDataTypeStr=boolean  SaturateOnIntegerOverflow=off  RndMeth=Floor
  MATLAB System : MATLABSystem  System=tfv_latch  SimulateUsing=Code generation
      mask Type: tfv_latch
      mask Display:
      | disp('tfv_latch');
      | port_label('input',1,'input');
      | port_label('input',2,'assert_lim');
      | port_label('input',3,'assert_vld');
      | port_label('input',4,'deassert_lim');
      | port_label('input',5,'deassert_vld');
      | port_label('input',6,'tmr');
      | port_label('output',1,'status');
  tfv_iphaseb : Outport  OutDataTypeStr=boolean
  wires:
  Data Type Conversion/1 -> tfv_iphaseb/1
  Data Store Read/1 -> MATLAB System/6
  deassert_vld/1 -> MATLAB System/5
  deassert_lim/1 -> MATLAB System/4
  assert_vld/1 -> MATLAB System/3
  assert_lim/1 -> MATLAB System/2
  input/1 -> MATLAB System/1
  MATLAB System/1 -> Data Type Conversion/1

== system npc_controller/IDLE_AND_TIMER/codegen/IDLE/idle_task1/hkeep/tfv/hkeep1/HKEEP.tfvIphaseC ==
  input : Inport  OutDataTypeStr=uint16  PortDimensions=1
  assert_lim : Inport  Port=2  OutDataTypeStr=uint16  PortDimensions=1
  assert_vld : Inport  Port=3  OutDataTypeStr=uint16  PortDimensions=1
  deassert_lim : Inport  Port=4  OutDataTypeStr=uint16  PortDimensions=1
  deassert_vld : Inport  Port=5  OutDataTypeStr=uint16  PortDimensions=1
  f : TriggerPort  TriggerType=function-call  VariantControl=(inherit)
      settings: CopyFcn=Stateflow.SLINSF.SimulinkMan.removeBlockPreDeleteFcn  PreDeleteFcn=Stateflow.SLINSF.SimulinkMan.unsafePredeleteFcn
  Data Store Read : DataStoreRead  DataStoreName=cnt_1ms  IndexOptions=Index vector (dialog)  Indices=1  OutputSizes=1
  Data Type Conversion : DataTypeConversion  OutDataTypeStr=boolean  SaturateOnIntegerOverflow=off  RndMeth=Floor
  MATLAB System : MATLABSystem  System=tfv_latch  SimulateUsing=Code generation
      mask Type: tfv_latch
      mask Display:
      | disp('tfv_latch');
      | port_label('input',1,'input');
      | port_label('input',2,'assert_lim');
      | port_label('input',3,'assert_vld');
      | port_label('input',4,'deassert_lim');
      | port_label('input',5,'deassert_vld');
      | port_label('input',6,'tmr');
      | port_label('output',1,'status');
  tfv_iphasec : Outport  OutDataTypeStr=boolean
  wires:
  Data Type Conversion/1 -> tfv_iphasec/1
  Data Store Read/1 -> MATLAB System/6
  deassert_vld/1 -> MATLAB System/5
  deassert_lim/1 -> MATLAB System/4
  assert_vld/1 -> MATLAB System/3
  assert_lim/1 -> MATLAB System/2
  input/1 -> MATLAB System/1
  MATLAB System/1 -> Data Type Conversion/1

== system npc_controller/IDLE_AND_TIMER/codegen/IDLE/idle_task1/hkeep/tfv/hkeep1/HKEEP.tfvVa ==
  input : Inport  OutDataTypeStr=uint16  PortDimensions=1
  assert_lim : Inport  Port=2  OutDataTypeStr=uint16  PortDimensions=1
  assert_vld : Inport  Port=3  OutDataTypeStr=uint16  PortDimensions=1
  deassert_lim : Inport  Port=4  OutDataTypeStr=uint16  PortDimensions=1
  deassert_vld : Inport  Port=5  OutDataTypeStr=uint16  PortDimensions=1
  f : TriggerPort  TriggerType=function-call  VariantControl=(inherit)
      settings: CopyFcn=Stateflow.SLINSF.SimulinkMan.removeBlockPreDeleteFcn  PreDeleteFcn=Stateflow.SLINSF.SimulinkMan.unsafePredeleteFcn
  Data Store Read : DataStoreRead  DataStoreName=cnt_1ms  IndexOptions=Index vector (dialog)  Indices=1  OutputSizes=1
  Data Type Conversion : DataTypeConversion  OutDataTypeStr=boolean  SaturateOnIntegerOverflow=off  RndMeth=Floor
  MATLAB System : MATLABSystem  System=tfv_latch  SimulateUsing=Code generation
      mask Type: tfv_latch
      mask Display:
      | disp('tfv_latch');
      | port_label('input',1,'input');
      | port_label('input',2,'assert_lim');
      | port_label('input',3,'assert_vld');
      | port_label('input',4,'deassert_lim');
      | port_label('input',5,'deassert_vld');
      | port_label('input',6,'tmr');
      | port_label('output',1,'status');
  tfv_va : Outport  OutDataTypeStr=boolean
  wires:
  Data Type Conversion/1 -> tfv_va/1
  Data Store Read/1 -> MATLAB System/6
  deassert_vld/1 -> MATLAB System/5
  deassert_lim/1 -> MATLAB System/4
  assert_vld/1 -> MATLAB System/3
  assert_lim/1 -> MATLAB System/2
  input/1 -> MATLAB System/1
  MATLAB System/1 -> Data Type Conversion/1

== system npc_controller/IDLE_AND_TIMER/codegen/IDLE/idle_task1/hkeep/tfv/hkeep1/HKEEP.tfvVaux ==
  input : Inport  OutDataTypeStr=uint16  PortDimensions=1
  assert_lim : Inport  Port=2  OutDataTypeStr=uint16  PortDimensions=1
  assert_vld : Inport  Port=3  OutDataTypeStr=uint16  PortDimensions=1
  deassert_lim : Inport  Port=4  OutDataTypeStr=uint16  PortDimensions=1
  deassert_vld : Inport  Port=5  OutDataTypeStr=uint16  PortDimensions=1
  f : TriggerPort  TriggerType=function-call  VariantControl=(inherit)
      settings: CopyFcn=Stateflow.SLINSF.SimulinkMan.removeBlockPreDeleteFcn  PreDeleteFcn=Stateflow.SLINSF.SimulinkMan.unsafePredeleteFcn
  Data Store Read : DataStoreRead  DataStoreName=cnt_1ms  IndexOptions=Index vector (dialog)  Indices=1  OutputSizes=1
  Data Type Conversion : DataTypeConversion  OutDataTypeStr=boolean  SaturateOnIntegerOverflow=off  RndMeth=Floor
  MATLAB System : MATLABSystem  System=tfv_latch  SimulateUsing=Code generation
      mask Type: tfv_latch
      mask Display:
      | disp('tfv_latch');
      | port_label('input',1,'input');
      | port_label('input',2,'assert_lim');
      | port_label('input',3,'assert_vld');
      | port_label('input',4,'deassert_lim');
      | port_label('input',5,'deassert_vld');
      | port_label('input',6,'tmr');
      | port_label('output',1,'status');
  Rate Transition2 : RateTransition  Commented=on
  tfv_vaux : Outport  OutDataTypeStr=boolean
  wires:
  Data Type Conversion/1 -> tfv_vaux/1
  deassert_vld/1 -> MATLAB System/5
  deassert_lim/1 -> MATLAB System/4
  assert_vld/1 -> MATLAB System/3
  assert_lim/1 -> MATLAB System/2
  input/1 -> MATLAB System/1
  MATLAB System/1 -> Data Type Conversion/1
  Data Store Read/1 -> MATLAB System/6

== system npc_controller/IDLE_AND_TIMER/codegen/IDLE/idle_task1/hkeep/tfv/hkeep1/HKEEP.tfvVb ==
  input : Inport  OutDataTypeStr=uint16  PortDimensions=1
  assert_lim : Inport  Port=2  OutDataTypeStr=uint16  PortDimensions=1
  assert_vld : Inport  Port=3  OutDataTypeStr=uint16  PortDimensions=1
  deassert_lim : Inport  Port=4  OutDataTypeStr=uint16  PortDimensions=1
  deassert_vld : Inport  Port=5  OutDataTypeStr=uint16  PortDimensions=1
  f : TriggerPort  TriggerType=function-call  VariantControl=(inherit)
      settings: CopyFcn=Stateflow.SLINSF.SimulinkMan.removeBlockPreDeleteFcn  PreDeleteFcn=Stateflow.SLINSF.SimulinkMan.unsafePredeleteFcn
  Data Store Read : DataStoreRead  DataStoreName=cnt_1ms  IndexOptions=Index vector (dialog)  Indices=1  OutputSizes=1
  Data Type Conversion : DataTypeConversion  OutDataTypeStr=boolean  SaturateOnIntegerOverflow=off  RndMeth=Floor
  MATLAB System : MATLABSystem  System=tfv_latch  SimulateUsing=Code generation
      mask Type: tfv_latch
      mask Display:
      | disp('tfv_latch');
      | port_label('input',1,'input');
      | port_label('input',2,'assert_lim');
      | port_label('input',3,'assert_vld');
      | port_label('input',4,'deassert_lim');
      | port_label('input',5,'deassert_vld');
      | port_label('input',6,'tmr');
      | port_label('output',1,'status');
  tfv_vb : Outport  OutDataTypeStr=boolean
  wires:
  Data Type Conversion/1 -> tfv_vb/1
  Data Store Read/1 -> MATLAB System/6
  deassert_vld/1 -> MATLAB System/5
  deassert_lim/1 -> MATLAB System/4
  assert_vld/1 -> MATLAB System/3
  assert_lim/1 -> MATLAB System/2
  input/1 -> MATLAB System/1
  MATLAB System/1 -> Data Type Conversion/1

== system npc_controller/IDLE_AND_TIMER/codegen/IDLE/idle_task1/hkeep/tfv/hkeep1/HKEEP.tfvVbulk ==
  input : Inport  OutDataTypeStr=uint16  PortDimensions=1
  assert_lim : Inport  Port=2  OutDataTypeStr=uint16  PortDimensions=1
  assert_vld : Inport  Port=3  OutDataTypeStr=uint16  PortDimensions=1
  deassert_lim : Inport  Port=4  OutDataTypeStr=uint16  PortDimensions=1
  deassert_vld : Inport  Port=5  OutDataTypeStr=uint16  PortDimensions=1
  f : TriggerPort  TriggerType=function-call  VariantControl=(inherit)
      settings: CopyFcn=Stateflow.SLINSF.SimulinkMan.removeBlockPreDeleteFcn  PreDeleteFcn=Stateflow.SLINSF.SimulinkMan.unsafePredeleteFcn
  Data Store Read : DataStoreRead  DataStoreName=cnt_1ms  IndexOptions=Index vector (dialog)  Indices=1  OutputSizes=1
  Data Type Conversion : DataTypeConversion  OutDataTypeStr=boolean  SaturateOnIntegerOverflow=off  RndMeth=Floor
  MATLAB System : MATLABSystem  System=tfv_latch  SimulateUsing=Code generation
      mask Type: tfv_latch
      mask Display:
      | disp('tfv_latch');
      | port_label('input',1,'input');
      | port_label('input',2,'assert_lim');
      | port_label('input',3,'assert_vld');
      | port_label('input',4,'deassert_lim');
      | port_label('input',5,'deassert_vld');
      | port_label('input',6,'tmr');
      | port_label('output',1,'status');
  tfv_vbulk : Outport  OutDataTypeStr=boolean
  wires:
  Data Type Conversion/1 -> tfv_vbulk/1
  Data Store Read/1 -> MATLAB System/6
  deassert_vld/1 -> MATLAB System/5
  deassert_lim/1 -> MATLAB System/4
  assert_vld/1 -> MATLAB System/3
  assert_lim/1 -> MATLAB System/2
  input/1 -> MATLAB System/1
  MATLAB System/1 -> Data Type Conversion/1

== system npc_controller/IDLE_AND_TIMER/codegen/IDLE/idle_task1/hkeep/tfv/hkeep1/HKEEP.tfvVc ==
  input : Inport  OutDataTypeStr=uint16  PortDimensions=1
  assert_lim : Inport  Port=2  OutDataTypeStr=uint16  PortDimensions=1
  assert_vld : Inport  Port=3  OutDataTypeStr=uint16  PortDimensions=1
  deassert_lim : Inport  Port=4  OutDataTypeStr=uint16  PortDimensions=1
  deassert_vld : Inport  Port=5  OutDataTypeStr=uint16  PortDimensions=1
  f : TriggerPort  TriggerType=function-call  VariantControl=(inherit)
      settings: CopyFcn=Stateflow.SLINSF.SimulinkMan.removeBlockPreDeleteFcn  PreDeleteFcn=Stateflow.SLINSF.SimulinkMan.unsafePredeleteFcn
  Data Store Read : DataStoreRead  DataStoreName=cnt_1ms  IndexOptions=Index vector (dialog)  Indices=1  OutputSizes=1
  Data Type Conversion : DataTypeConversion  OutDataTypeStr=boolean  SaturateOnIntegerOverflow=off  RndMeth=Floor
  MATLAB System : MATLABSystem  System=tfv_latch  SimulateUsing=Code generation
      mask Type: tfv_latch
      mask Display:
      | disp('tfv_latch');
      | port_label('input',1,'input');
      | port_label('input',2,'assert_lim');
      | port_label('input',3,'assert_vld');
      | port_label('input',4,'deassert_lim');
      | port_label('input',5,'deassert_vld');
      | port_label('input',6,'tmr');
      | port_label('output',1,'status');
  tfv_vc : Outport  OutDataTypeStr=boolean
  wires:
  Data Type Conversion/1 -> tfv_vc/1
  Data Store Read/1 -> MATLAB System/6
  deassert_vld/1 -> MATLAB System/5
  deassert_lim/1 -> MATLAB System/4
  assert_vld/1 -> MATLAB System/3
  assert_lim/1 -> MATLAB System/2
  input/1 -> MATLAB System/1
  MATLAB System/1 -> Data Type Conversion/1

== system npc_controller/IDLE_AND_TIMER/codegen/IDLE/idle_task1/hkeep/tfv/hkeep1/HKEEP.tfvVmid ==
  input : Inport  OutDataTypeStr=uint16  PortDimensions=1
  assert_lim : Inport  Port=2  OutDataTypeStr=uint16  PortDimensions=1
  assert_vld : Inport  Port=3  OutDataTypeStr=uint16  PortDimensions=1
  deassert_lim : Inport  Port=4  OutDataTypeStr=uint16  PortDimensions=1
  deassert_vld : Inport  Port=5  OutDataTypeStr=uint16  PortDimensions=1
  f : TriggerPort  TriggerType=function-call  VariantControl=(inherit)
      settings: CopyFcn=Stateflow.SLINSF.SimulinkMan.removeBlockPreDeleteFcn  PreDeleteFcn=Stateflow.SLINSF.SimulinkMan.unsafePredeleteFcn
  Data Store Read : DataStoreRead  DataStoreName=cnt_1ms  IndexOptions=Index vector (dialog)  Indices=1  OutputSizes=1
  Data Type Conversion : DataTypeConversion  OutDataTypeStr=boolean  SaturateOnIntegerOverflow=off  RndMeth=Floor
  MATLAB System : MATLABSystem  System=tfv_latch  SimulateUsing=Code generation
      mask Type: tfv_latch
      mask Display:
      | disp('tfv_latch');
      | port_label('input',1,'input');
      | port_label('input',2,'assert_lim');
      | port_label('input',3,'assert_vld');
      | port_label('input',4,'deassert_lim');
      | port_label('input',5,'deassert_vld');
      | port_label('input',6,'tmr');
      | port_label('output',1,'status');
  Rate Transition2 : RateTransition  Commented=on
  tfv_vmid : Outport  OutDataTypeStr=boolean
  wires:
  Data Type Conversion/1 -> tfv_vmid/1
  deassert_vld/1 -> MATLAB System/5
  deassert_lim/1 -> MATLAB System/4
  assert_vld/1 -> MATLAB System/3
  assert_lim/1 -> MATLAB System/2
  input/1 -> MATLAB System/1
  MATLAB System/1 -> Data Type Conversion/1
  Data Store Read/1 -> MATLAB System/6

== system npc_controller/IDLE_AND_TIMER/codegen/IDLE/idle_task1/hkeep/tz/System Outputs2 ==

== system npc_controller/IDLE_AND_TIMER/codegen/IDLE/idle_task1/set_tmp_mux/incr_cnt_tmp_mux/cnt_idle ==
  Action Port : ActionPort  ActionPortLabel=if(u1 < 4)
  Add : Sum
  Constant : Constant  OutDataTypeStr=uint16
  Data Store Read1 : DataStoreRead  DataStoreName=cnt_tmp_mux  IndexOptions=Index vector (dialog)  Indices=1  OutputSizes=1
  Data Store Write : DataStoreWrite  DataStoreName=cnt_tmp_mux  IndexOptions=Index vector (dialog)  Indices=1  OutputSizes=1
  wires:
  Data Store Read1/1 -> Add/1
  Add/1 -> Data Store Write/1
  Constant/1 -> Add/2

== system npc_controller/IDLE_AND_TIMER/codegen/IDLE/idle_task1/set_tmp_mux/incr_cnt_tmp_mux/cnt_idle_sat ==
  Action Port : ActionPort  ActionPortLabel=else
  Constant : Constant  Value=0  OutDataTypeStr=uint16
  Data Store Write : DataStoreWrite  DataStoreName=cnt_tmp_mux  IndexOptions=Index vector (dialog)  Indices=1  OutputSizes=1
  wires:
  Constant/1 -> Data Store Write/1

== system npc_controller/IDLE_AND_TIMER/codegen/IDLE/idle_task1/set_tmp_mux/parse_cnt_tmp_mux/cnt_tmp_mux_0 ==
  Action Port : ActionPort  ActionPortLabel=case [ 0 ]:
  Constant : Constant  Value=0  OutDataTypeStr=boolean  SampleTime=-1
  Constant1 : Constant  Value=0  OutDataTypeStr=boolean  SampleTime=-1
  Constant2 : Constant  Value=0  OutDataTypeStr=boolean  SampleTime=-1
  Data Store Write : DataStoreWrite  DataStoreName=tmp_mux_s0  IndexOptions=Index vector (dialog)  Indices=1  OutputSizes=1
  Data Store Write1 : DataStoreWrite  DataStoreName=tmp_mux_s1  IndexOptions=Index vector (dialog)  Indices=1  OutputSizes=1
  Data Store Write2 : DataStoreWrite  DataStoreName=tmp_mux_s2  IndexOptions=Index vector (dialog)  Indices=1  OutputSizes=1
  wires:
  Constant/1 -> Data Store Write/1
  Constant1/1 -> Data Store Write1/1
  Constant2/1 -> Data Store Write2/1

== system npc_controller/IDLE_AND_TIMER/codegen/IDLE/idle_task1/set_tmp_mux/parse_cnt_tmp_mux/cnt_tmp_mux_1 ==
  Action Port : ActionPort  ActionPortLabel=case [ 1 ]:
  Constant : Constant  OutDataTypeStr=boolean  SampleTime=-1
  Constant1 : Constant  Value=0  OutDataTypeStr=boolean  SampleTime=-1
  Constant2 : Constant  Value=0  OutDataTypeStr=boolean  SampleTime=-1
  Data Store Write : DataStoreWrite  DataStoreName=tmp_mux_s0  IndexOptions=Index vector (dialog)  Indices=1  OutputSizes=1
  Data Store Write1 : DataStoreWrite  DataStoreName=tmp_mux_s1  IndexOptions=Index vector (dialog)  Indices=1  OutputSizes=1
  Data Store Write2 : DataStoreWrite  DataStoreName=tmp_mux_s2  IndexOptions=Index vector (dialog)  Indices=1  OutputSizes=1
  wires:
  Constant2/1 -> Data Store Write2/1
  Constant1/1 -> Data Store Write1/1
  Constant/1 -> Data Store Write/1

== system npc_controller/IDLE_AND_TIMER/codegen/IDLE/idle_task1/set_tmp_mux/parse_cnt_tmp_mux/cnt_tmp_mux_2 ==
  Action Port : ActionPort  ActionPortLabel=case [ 2 ]:
  Constant : Constant  Value=0  OutDataTypeStr=boolean  SampleTime=-1
  Constant1 : Constant  OutDataTypeStr=boolean  SampleTime=-1
  Constant2 : Constant  Value=0  OutDataTypeStr=boolean  SampleTime=-1
  Data Store Write : DataStoreWrite  DataStoreName=tmp_mux_s0  IndexOptions=Index vector (dialog)  Indices=1  OutputSizes=1
  Data Store Write1 : DataStoreWrite  DataStoreName=tmp_mux_s1  IndexOptions=Index vector (dialog)  Indices=1  OutputSizes=1
  Data Store Write2 : DataStoreWrite  DataStoreName=tmp_mux_s2  IndexOptions=Index vector (dialog)  Indices=1  OutputSizes=1
  wires:
  Constant/1 -> Data Store Write/1
  Constant1/1 -> Data Store Write1/1
  Constant2/1 -> Data Store Write2/1

== system npc_controller/IDLE_AND_TIMER/codegen/IDLE/idle_task1/set_tmp_mux/parse_cnt_tmp_mux/cnt_tmp_mux_3 ==
  Action Port : ActionPort  ActionPortLabel=case [ 3 ]:
  Constant : Constant  OutDataTypeStr=boolean  SampleTime=-1
  Constant1 : Constant  OutDataTypeStr=boolean  SampleTime=-1
  Constant2 : Constant  Value=0  OutDataTypeStr=boolean  SampleTime=-1
  Data Store Write : DataStoreWrite  DataStoreName=tmp_mux_s0  IndexOptions=Index vector (dialog)  Indices=1  OutputSizes=1
  Data Store Write1 : DataStoreWrite  DataStoreName=tmp_mux_s1  IndexOptions=Index vector (dialog)  Indices=1  OutputSizes=1
  Data Store Write2 : DataStoreWrite  DataStoreName=tmp_mux_s2  IndexOptions=Index vector (dialog)  Indices=1  OutputSizes=1
  wires:
  Constant2/1 -> Data Store Write2/1
  Constant1/1 -> Data Store Write1/1
  Constant/1 -> Data Store Write/1

== system npc_controller/CONTROL/CONTROL/false/CLA_CONTROL/CONTROL/pwm_generation1/Subsystem/If Action Subsystem ==
  In1 : Inport
  Action Port : ActionPort  ActionPortLabel=if(u1 == 0)
  Out1 : Outport
  wires:
  In1/1 -> Out1/1

== system npc_controller/CONTROL/CONTROL/false/CLA_CONTROL/CONTROL/pwm_generation1/Subsystem/If Action Subsystem1 ==
  In1 : Inport
  Action Port : ActionPort  ActionPortLabel=else
  Out1 : Outport
  wires:
  In1/1 -> Out1/1

== system npc_controller/CONTROL/CONTROL/false/CLA_CONTROL/CONTROL/pwm_generation1/Subsystem1/If Action Subsystem ==
  In1 : Inport
  Action Port : ActionPort  ActionPortLabel=if(u1 == 0)
  Out1 : Outport
  wires:
  In1/1 -> Out1/1

== system npc_controller/CONTROL/CONTROL/false/CLA_CONTROL/CONTROL/pwm_generation1/Subsystem1/If Action Subsystem1 ==
  In1 : Inport
  Action Port : ActionPort  ActionPortLabel=else
  Out1 : Outport
  wires:
  In1/1 -> Out1/1

== system npc_controller/CONTROL/CONTROL/false/CLA_CONTROL/CONTROL/pwm_generation1/Subsystem2/If Action Subsystem ==
  In1 : Inport
  Action Port : ActionPort  ActionPortLabel=if(u1 == 0)
  Out1 : Outport
  wires:
  In1/1 -> Out1/1

== system npc_controller/CONTROL/CONTROL/false/CLA_CONTROL/CONTROL/pwm_generation1/Subsystem2/If Action Subsystem1 ==
  In1 : Inport
  Action Port : ActionPort  ActionPortLabel=else
  Out1 : Outport
  wires:
  In1/1 -> Out1/1

== system npc_controller/CONTROL/CONTROL/false/CLA_CONTROL/CONTROL/pwm_generation1/min_duty/Duty0Pct ==
  Action Port : ActionPort  ActionPortLabel=else
  Constant : Constant  Value=0  OutDataTypeStr=single  SampleTime=-1
  Out1 : Outport
  wires:
  Constant/1 -> Out1/1

== system npc_controller/CONTROL/CONTROL/false/CLA_CONTROL/CONTROL/pwm_generation1/min_duty/Duty5Pct ==
  In1 : Inport
  Action Port : ActionPort  ActionPortLabel=if(u1 > 76)
  Out1 : Outport
  wires:
  In1/1 -> Out1/1
